simulink model "fp_simulink_model"  (Simulink 7.8)
settings: Solver=VariableStepDiscrete  StartTime=0.0  StopTime=10.0  RelTol=1e-3
undefined symbols (not defined in the file or in its folder): BitWidth
libraries: vmodel_blocks x1
settings Model: Creator=chuh  LastModifiedBy=chuh

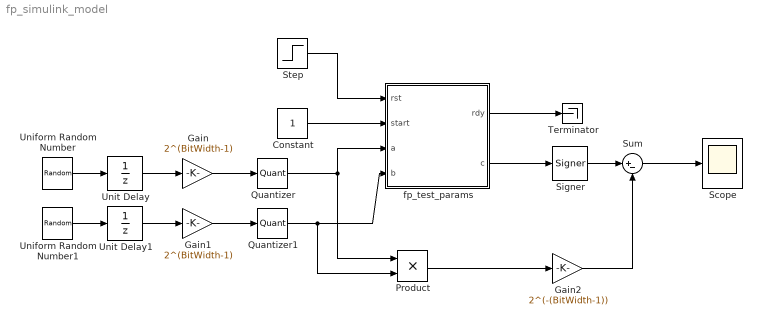
== system fp_simulink_model ==
  Constant : Constant
  Gain : Gain  Gain=2^(BitWidth-1)
  Gain1 : Gain  Gain=2^(BitWidth-1)
  Gain2 : Gain  Gain=2^(-(BitWidth-1))
  Product : Product  RndMeth=Zero
  Quantizer : Quantizer  QuantizationInterval=1
  Quantizer1 : Quantizer  QuantizationInterval=1
  Scope : Scope
      settings: YMin=-7  YMax=10  SaveName=sim_error  SampleInput=on  SampleTime=0.001
  Signer : vmodel_blocks/Signer  N=BitWidth
  Step : Step  Time=0.002  Before=1  After=0  SampleTime=0
  Sum : Sum  Inputs=|+-
  Terminator : Terminator
  Uniform Random Number : UniformRandomNumber  Maximum=0.99999  SampleTime=0.001
  Uniform Random Number1 : UniformRandomNumber  Maximum=0.99999  Seed=2435324  SampleTime=0.001
  Unit Delay : UnitDelay  SampleTime=0.002
  Unit Delay1 : UnitDelay  SampleTime=0.002
  fp_test_params : Subsystem  mask(fp_test_params){params_samples=0.001, params_freq=50}
      mask prompts: params_samples "Sample time:"; params_freq "FPGA frequency (MHz):"
      mask help:
      | input rst
      | input start
      | input a[15:0]
      | input b[15:0]
      | output rdy
      | output c[15:0]
      mask Help:
      | input rst
      | input start
      | input a[15:0]
      | input b[15:0]
      | output rdy
      | output c[15:0]
  wires:
  Constant/1 -> fp_test_params/2(start)
  Step/1 -> fp_test_params/1(rst)
  Uniform Random Number/1 -> Unit Delay/1
  Uniform Random Number1/1 -> Unit Delay1/1
  Gain/1 -> Quantizer/1
  Gain1/1 -> Quantizer1/1
  fp_test_params/2(c) -> Signer/1
  Sum/1 -> Scope/1
  Product/1 -> Gain2/1
  Signer/1 -> Sum/1
  Gain2/1 -> Sum/2
  Unit Delay/1 -> Gain/1
  Unit Delay1/1 -> Gain1/1
  fp_test_params/1(rdy) -> Terminator/1
  Quantizer/1 -> fp_test_params/3(a), Product/1
  Quantizer1/1 -> fp_test_params/4(b), Product/2

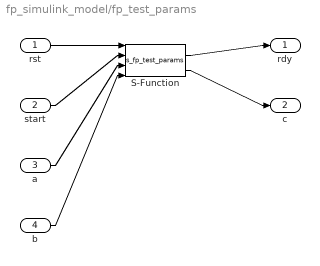
== system fp_simulink_model/fp_test_params ==
  rst : Inport  OutDataTypeStr=double  SampleTime=0.001
  start : Inport  Port=2  OutDataTypeStr=double  SampleTime=0.001
  a : Inport  Port=3  OutDataTypeStr=double  SampleTime=0.001
  b : Inport  Port=4  OutDataTypeStr=double  SampleTime=0.001
  S-Function : S-Function  FunctionName=s_fp_test_params  Parameters=params_samples, params_freq  EnableBusSupport=off
  rdy : Outport  OutDataTypeStr=uint32  SampleTime=0.001
  c : Outport  Port=2  OutDataTypeStr=uint32  SampleTime=0.001
  wires:
  rst/1 -> S-Function/1
  start/1 -> S-Function/2
  a/1 -> S-Function/3
  b/1 -> S-Function/4
  S-Function/1 -> rdy/1
  S-Function/2 -> c/1
